simulink model "verify"  (R2017b)
settings: Solver=ode14x  StartTime=0.0  StopTime=10.0  FixedStep=0.01  RelTol=1e-3
settings Model: Creator=lenovo  LastModifiedBy=lenovo

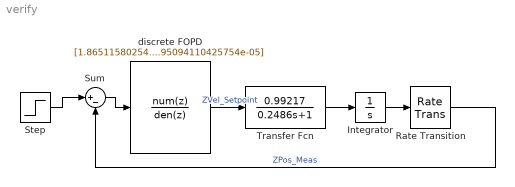
== system verify ==
  Integrator : Integrator
  Rate Transition : RateTransition  OutPortSampleTime=0.01
  Step : Step  SampleTime=0.01
  Sum : Sum  Inputs=|+-
  Transfer Fcn : TransferFcn  Numerator=[0.99217]  Denominator=[0.2486 1]
  discrete FOPD : DiscreteTransferFcn  Numerator=[1.86511580254824,-6.20360416522752,7.77951053722034,-4.47930158754086,1.12529607747831,-0.0867420445559554]  Denominator=[0.0101201839324044,-0.0228427827690589,0.0162967440497079,-0.00320636053105791,-0.000423005899049262,8.95094110425754e-05]  SampleTime=0.01
  wires:
  Step/1 -> Sum/1
  Sum/1 -> discrete FOPD/1
  discrete FOPD/1 -> Transfer Fcn/1  "ZVel_Setpoint"
  Transfer Fcn/1 -> Integrator/1
  Integrator/1 -> Rate Transition/1
  Rate Transition/1 -> Sum/2  "ZPos_Meas"
